simulink model "BIM_3phaseModel_MidInject_DPNV"  (R2022b)
settings: Solver=VariableStepAuto  StartTime=0.0  StopTime=3  RelTol=1e-3
values from neighbouring files (symbols this model uses):
  Ad_s1_s = 0.730402691048646    (= 0.730402691049)    [BIM_init.m]
  Ad_t_s = 0.881911378298176    (= 0.881911378298)    [BIM_init.m]
  Ap_s1_s = 0.975904794542392    (= 0.975904794542)    [BIM_init.m]
  Ap_t_s = 0.995669127615556    (= 0.995669127616)    [BIM_init.m]
  Bd_s1_s = 0.269597308951354    (= 0.269597308951)    [BIM_init.m]
  Bd_t_s = 0.118088621701824    (= 0.118088621702)    [BIM_init.m]
  Bp_s1_s = 0.269597308951354    (= 0.269597308951)    [BIM_init.m]
  Bp_t_s = 0.118088621701824    (= 0.118088621702)    [BIM_init.m]
  Ctr_v_Ki = Ctr_v_Kp*0.1    (= 0.1)    [BIM_init.m]
  Ctr_v_Kp = 1    [BIM_init.m]
  L_m = 5.02e-3    (= 0.00502)    [BIM_init.m]
  L_r = L_m + L_sigma_r    (= 0.00576)    [BIM_init.m]
  m_rotor = 1.5    [BIM_init.m]
  PolePair = 1    [BIM_init.m]
  r_s1_s = 2*R_s    (= 1)    [BIM_init.m]
  r_t_s = R_s/2    (= 0.25)    [BIM_init.m]
  T = 1/fsw    (= 0.0001)    [BIM_init.m]
  tau_r = 0.012255319148936    (= 0.0122553191489)    [BIM_init.m]
  Ts = 1/fsw    (= 0.0001)    [BIM_init.m]
undefined symbols (not defined in the file or in its folder): plecs, sigbuilder_block
libraries: spsabctodq0Lib x8, spsdq0toabcLib x4
(part 1 of 2)
settings Model: Creator=Zhouzhou  LastModifiedBy=Zhouzhou
settings SolverCC: AlgebraicLoopSolver=TrustRegion
settings DebuggingCC: UnconnectedInputMsg=warning  UnconnectedOutputMsg=warning  UnconnectedLineMsg=warning  SFMachineParentedDataDiag=warning
settings ModelReferenceCC: EnableRefExpFcnMdlSchedulingChecks=on
settings RTWCC: DLArmComputeVersion=19.05

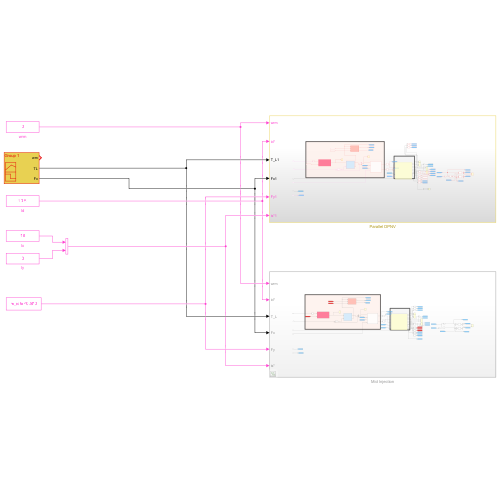
[thumbnail: Simulink's stored preview of the top-level diagram]
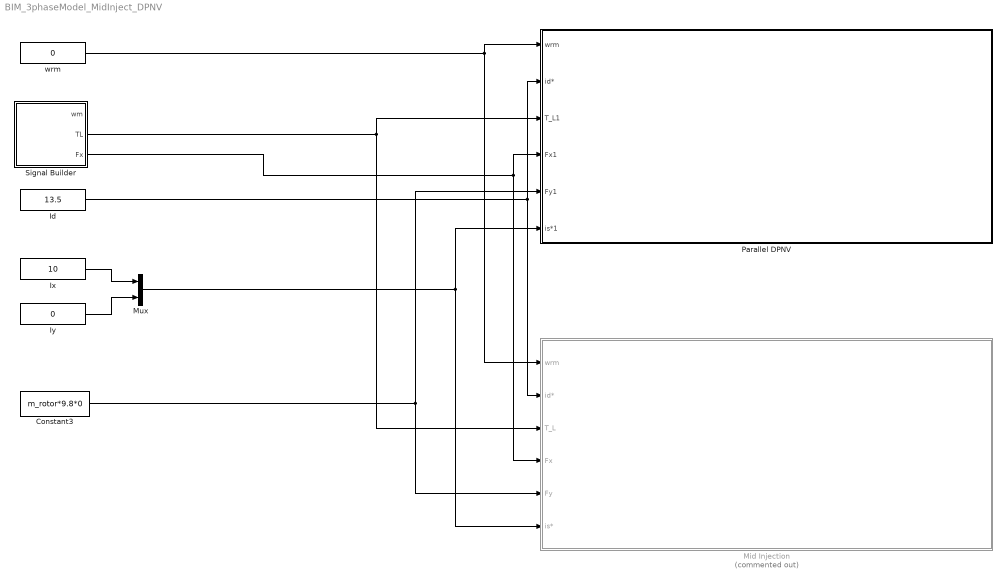
== system BIM_3phaseModel_MidInject_DPNV ==
  Constant3 : Constant  Value=m_rotor*9.8*0
  Id : Constant  Value=13.5
  Ix : Constant  Value=10
  Iy : Constant  Value=0
  Mid Injection : Subsystem  Commented=on
  Mux : Mux  Inputs=2
  Parallel DPNV : Subsystem
  Signal Builder : Subsystem  Tag=STV Subsys  LoadFcn=sigbuilder_block('load');  StartFcn=sigbuilder_block('start');  StopFcn=sigbuilder_block('stop');  ClipboardFcn=sigbuilder_block('clipboard');  mask(Sigbuilder block){tuvar=[0:10]}
      mask help: Simulink:masks:SigbuilderBlock_MD
      mask init:
      | if ~strcmp(get_param(bdroot(gcbh),'SimulationStatus'),'stopped') tuvar = sigbuilder_block('maskInit'); end
      settings: CopyFcn=sigbuilder_block('copy');  DeleteFcn=sigbuilder_block('delete');  ModelCloseFcn=sigbuilder_block('modelClose');  PreSaveFcn=sigbuilder_block('preSave');  PauseFcn=sigbuilder_block('pause');  ContinueFcn=sigbuilder_block('continue');  NameChangeFcn=sigbuilder_block('namechange');  OpenFcn=sigbuilder_block('open',[4.5 4.5 951 480.25 ]);  CloseFcn=sigbuilder_block('close');
      mask Display: plot(0, 0, 100, 100,[2, 2, 32, 32, 2], [68, 8, 8, 68, 68],[32, 2], [38, 38], [32, 19, 2],[53, 60, 44], [32, 17, 17, 2],[16, 16, 31, 31]);txt = getActiveGroup(gcbh);text(2, 100, txt,'verticalAlignment', 'top');
  wrm : Constant  Value=0
  wires:
  wrm/1 -> Mid Injection/1(wrm), Parallel DPNV/1(wrm)
  Signal Builder/2(TL) -> Parallel DPNV/3(T_L1), Mid Injection/3(T_L)
  Id/1 -> Parallel DPNV/2(id*), Mid Injection/2(id*)
  Constant3/1 -> Mid Injection/5(Fy), Parallel DPNV/5(Fy1)
  Signal Builder/3(Fx) -> Parallel DPNV/4(Fx1), Mid Injection/4(Fx)
  Ix/1 -> Mux/1
  Iy/1 -> Mux/2
  Mux/1 -> Mid Injection/6(is*), Parallel DPNV/6(is*1)

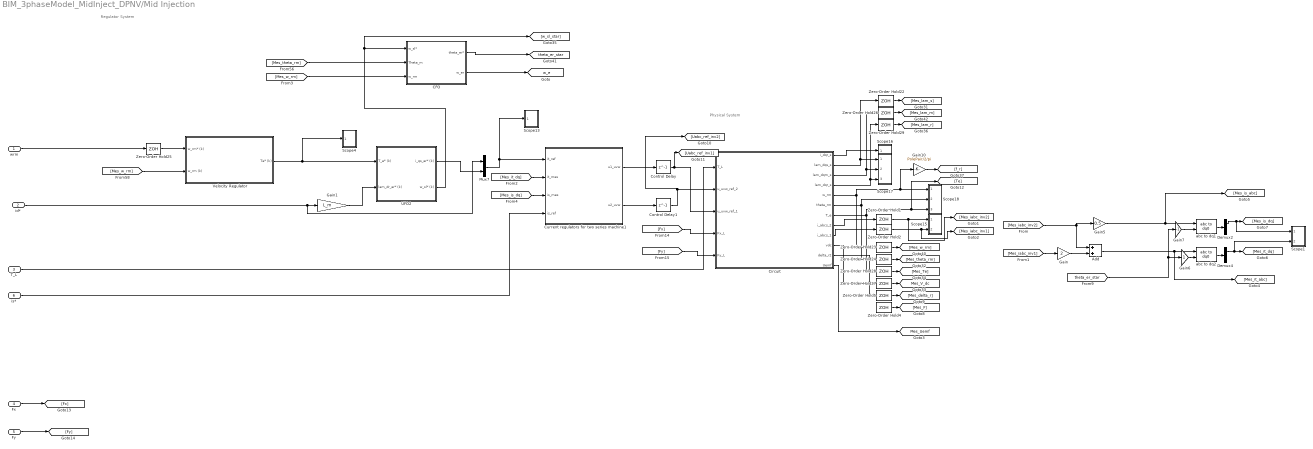
== system BIM_3phaseModel_MidInject_DPNV/Mid Injection ==
  note: Regulator System
  note: Physical System
  wrm : Inport
  id* : Inport  Port=2
  T_L : Inport  Port=3
  Fx : Inport  Port=4
  Fy : Inport  Port=5
  is* : Inport  Port=6
  Add : Sum
  CFO : Subsystem
  Circuit : Subsystem  LoadFcn=plecs('sl', 200);  InitFcn=plecs('sl', 214);  StartFcn=plecs('sl', 208);  StopFcn=plecs('sl', 209);  mask(PlecsCircuit){PLECSData=<binary blob, 27032 chars, not shown>}
      mask prompts: PLECSData "PLECS Data (Do not delete or modify!)"
      mask init:
      | % PLACE CUSTOM INITIALIZATIONS ABOVE
      | % DO NOT REMOVE
      | plecs('sl', 215);
      | % DO NOT REMOVE
      settings: CopyFcn=plecs('sl', 203);  DeleteFcn=plecs('sl', 205);  UndoDeleteFcn=plecs('sl', 206);  PreSaveFcn=plecs('sl', 211);  PostSaveFcn=plecs('sl', 201);  NameChangeFcn=plecs('sl', 210);  DestroyFcn=plecs('sl', 207);  PreCopyFcn=plecs('sl', 216);  OpenFcn=plecs('sl', 202);  ErrorFcn=plerrorfcn
      mask Help: web(['file:///' fullfile(plecsdoc, 'creatingacircuit.html')])
      mask Display: disp('IM Drive System');
  Control Delay : Delay  DelayLength=1  InitialCondition=0  SampleTime=T
  Control Delay1 : Delay  DelayLength=1  InitialCondition=0  SampleTime=T
  Current regulators for two series machine1 : Subsystem
  Demux2 : Demux  Outputs=[2 1]
  Demux4 : Demux  Outputs=[2 1]
  Gain : Gain  Gain=2
  Gain1 : Gain  Gain=L_m
  Gain10 : Gain  Gain=PolePair/2/pi
  Gain5 : Gain  Gain=0.5
  Gain6 : Gain
  Gain7 : Gain  Gain=-1
  Mux7 : Mux  Inputs=2
  Scope1 : Subsystem  LoadFcn=plecs('sl', 300);  InitFcn=plecs('sl', 314);  StartFcn=plecs('sl', 308);  StopFcn=plecs('sl', 309);  mask{Settings=<binary blob, 232 chars, not shown>}
      mask init:
      | plecs('sl', 315);
      settings: CopyFcn=plecs('sl', 303);  DeleteFcn=plecs('sl', 305);  UndoDeleteFcn=plecs('sl', 306);  PreSaveFcn=plecs('sl', 311);  NameChangeFcn=plecs('sl', 310);  DestroyFcn=plecs('sl', 307);  OpenFcn=plecs('sl', 302);  ErrorFcn=plerrorfcn
      mask Display: plot([0.1 0.9 0.9 0.1 0.1], [0.9 0.9 0.5 0.5 0.9])
  Scope13 : Subsystem  LoadFcn=plecs('sl', 300);  InitFcn=plecs('sl', 314);  StartFcn=plecs('sl', 308);  StopFcn=plecs('sl', 309);  mask{Settings=<binary blob, 232 chars, not shown>}
      mask init:
      | plecs('sl', 315);
      settings: CopyFcn=plecs('sl', 303);  DeleteFcn=plecs('sl', 305);  UndoDeleteFcn=plecs('sl', 306);  PreSaveFcn=plecs('sl', 311);  NameChangeFcn=plecs('sl', 310);  DestroyFcn=plecs('sl', 307);  OpenFcn=plecs('sl', 302);  ErrorFcn=plerrorfcn
      mask Display: plot([0.1 0.9 0.9 0.1 0.1], [0.9 0.9 0.5 0.5 0.9])
  Scope15 : Subsystem  LoadFcn=plecs('sl', 300);  InitFcn=plecs('sl', 314);  StartFcn=plecs('sl', 308);  StopFcn=plecs('sl', 309);  mask{Settings=<binary blob, 232 chars, not shown>}
      mask init:
      | plecs('sl', 315);
      settings: CopyFcn=plecs('sl', 303);  DeleteFcn=plecs('sl', 305);  UndoDeleteFcn=plecs('sl', 306);  PreSaveFcn=plecs('sl', 311);  NameChangeFcn=plecs('sl', 310);  DestroyFcn=plecs('sl', 307);  OpenFcn=plecs('sl', 302);  ErrorFcn=plerrorfcn
      mask Display: plot([0.1 0.9 0.9 0.1 0.1], [0.9 0.9 0.5 0.5 0.9])
  Scope16 : Subsystem  LoadFcn=plecs('sl', 300);  InitFcn=plecs('sl', 314);  StartFcn=plecs('sl', 308);  StopFcn=plecs('sl', 309);  mask{Settings=<binary blob, 232 chars, not shown>}
      mask init:
      | plecs('sl', 315);
      settings: CopyFcn=plecs('sl', 303);  DeleteFcn=plecs('sl', 305);  UndoDeleteFcn=plecs('sl', 306);  PreSaveFcn=plecs('sl', 311);  NameChangeFcn=plecs('sl', 310);  DestroyFcn=plecs('sl', 307);  OpenFcn=plecs('sl', 302);  ErrorFcn=plerrorfcn
      mask Display: plot([0.1 0.9 0.9 0.1 0.1], [0.9 0.9 0.5 0.5 0.9])
  Scope17 : Subsystem  LoadFcn=plecs('sl', 300);  InitFcn=plecs('sl', 314);  StartFcn=plecs('sl', 308);  StopFcn=plecs('sl', 309);  mask{Settings=<binary blob, 232 chars, not shown>}
      mask init:
      | plecs('sl', 315);
      settings: CopyFcn=plecs('sl', 303);  DeleteFcn=plecs('sl', 305);  UndoDeleteFcn=plecs('sl', 306);  PreSaveFcn=plecs('sl', 311);  NameChangeFcn=plecs('sl', 310);  DestroyFcn=plecs('sl', 307);  OpenFcn=plecs('sl', 302);  ErrorFcn=plerrorfcn
      mask Display: plot([0.1 0.9 0.9 0.1 0.1], [0.9 0.9 0.5 0.5 0.9])
  Scope18 : Subsystem  LoadFcn=plecs('sl', 300);  InitFcn=plecs('sl', 314);  StartFcn=plecs('sl', 308);  StopFcn=plecs('sl', 309);  mask{Settings=<binary blob, 232 chars, not shown>}
      mask init:
      | plecs('sl', 315);
      settings: CopyFcn=plecs('sl', 303);  DeleteFcn=plecs('sl', 305);  UndoDeleteFcn=plecs('sl', 306);  PreSaveFcn=plecs('sl', 311);  NameChangeFcn=plecs('sl', 310);  DestroyFcn=plecs('sl', 307);  OpenFcn=plecs('sl', 302);  ErrorFcn=plerrorfcn
      mask Display: plot([0.1 0.9 0.9 0.1 0.1], [0.9 0.9 0.5 0.5 0.9])
  Scope4 : Subsystem  LoadFcn=plecs('sl', 300);  InitFcn=plecs('sl', 314);  StartFcn=plecs('sl', 308);  StopFcn=plecs('sl', 309);  mask{Settings=<binary blob, 232 chars, not shown>}
      mask init:
      | plecs('sl', 315);
      settings: CopyFcn=plecs('sl', 303);  DeleteFcn=plecs('sl', 305);  UndoDeleteFcn=plecs('sl', 306);  PreSaveFcn=plecs('sl', 311);  NameChangeFcn=plecs('sl', 310);  DestroyFcn=plecs('sl', 307);  OpenFcn=plecs('sl', 302);  ErrorFcn=plerrorfcn
      mask Display: plot([0.1 0.9 0.9 0.1 0.1], [0.9 0.9 0.5 0.5 0.9])
  UFO2 : Subsystem
  Velocity Regulator : Subsystem
  Zero-Order Hold{1..2,4..5,22..29} (12 alike) : ZeroOrderHold  SampleTime=T
  abc to dq1 : spsabctodq0Lib/abc to dq0  Alignment=Aligned with phase A axis
  abc to dq2 : spsabctodq0Lib/abc to dq0  Alignment=Aligned with phase A axis
  tag scope: Mes_Uemf=global, Mes_V_dc=global, theta_er_star=global, w_e=global
  wires:
  Zero-Order Hold22/1 -> [Mes_lam_s]
  Gain6/1 -> abc to dq2/2
  [theta_er_star] -> Gain7/1, Gain6/1
  [Mes_w_rm] -> CFO/3(w_rm)
  Circuit/5(w_rm) -> Scope18/1(1), Gain10/1, Zero-Order Hold23/1
  Zero-Order Hold29/1 -> [Mes_lam_r]
  Circuit/1(i_dqr_s) -> Scope16/1(1)
  Circuit/6(theta_rm) -> Scope18/2(2), Zero-Order Hold24/1
  CFO/1(theta_er*) -> [theta_er_star]
  Circuit/4(lam_dqr_s) -> Scope17/3(3), Zero-Order Hold29/1
  abc to dq1/1 -> Demux2/1
  Add/1 -> [Mes_it_abc], abc to dq2/1
  UFO2/2(w_sl* (k)) -> [w_sl_star], CFO/1(w_sl*)
  [Mes_iabc_inv1] -> Gain/1
  Demux4/1 -> Scope1/2(2), [Mes_it_dq]
  Mux7/1 -> Current regulators for two series machine1/1(it_ref), Scope13/1(1)
  [Fx] -> Circuit/4(Fx_L)
  [Mes_w_rm] -> Velocity Regulator/2(w_rm (k))
  Circuit/2(lam_dqs_s) -> Scope17/1(1), Zero-Order Hold22/1
  Circuit/7(T_e) -> [Te], Scope18/3(3), Zero-Order Hold28/1
  [Mes_theta_rm] -> CFO/2(Theta_m)
  Current regulators for two series machine1/1(u1_uvw) -> Control Delay/1
  Zero-Order Hold28/1 -> [Mes_Te]
  Gain10/1 -> [f_r]
  Zero-Order Hold4/1 -> [Mes_F]
  id*/1 -> Mux7/1, Gain1/1
  Zero-Order Hold2/1 -> [Mes_iabc_inv1], Scope15/2(2)
  [Mes_iabc_inv2] -> Gain5/1, Add/1
  Zero-Order Hold25/1 -> Velocity Regulator/1(w_rm* (k))
  Current regulators for two series machine1/2(u2_uvw) -> Control Delay1/1
  Gain1/1 -> UFO2/2(lam_dr_er* (k))
  Circuit/8(i_abcs_2) -> Zero-Order Hold1/1
  [Mes_is_dq] -> Current regulators for two series machine1/3(is_mes)
  Circuit/9(i_abcs_1) -> Zero-Order Hold2/1
  Gain/1 -> Add/2
  Zero-Order Hold1/1 -> [Mes_iabc_inv2], Scope15/1(1)
  Zero-Order Hold23/1 -> [Mes_w_rm]
  Demux2/1 -> Scope1/1(1), [Mes_is_dq]
  Circuit/11(delta_r2) -> Zero-Order Hold5/1
  abc to dq2/1 -> Demux4/1
  [Mes_it_dq] -> Current regulators for two series machine1/2(it_mes)
  Velocity Regulator/1(Te* (k)) -> Scope4/1(1), UFO2/1(T_e* (k))
  Zero-Order Hold24/1 -> [Mes_theta_rm]
  Zero-Order Hold26/1 -> [Mes_lam_m]
  Zero-Order Hold27/1 -> [Mes_V_dc]
  [Fy] -> Circuit/5(Fy_L)
  Circuit/10(vdc) -> Zero-Order Hold27/1
  Circuit/3(lam_dqm_s) -> Scope17/2(2), Zero-Order Hold26/1
  CFO/2(w_er) -> [w_e]
  UFO2/1(i_qs_er* (k)) -> Mux7/2
  Zero-Order Hold5/1 -> [Mes_delta_r]
  T_L/1 -> Circuit/1(T_L)
  wrm/1 -> Zero-Order Hold25/1
  Control Delay1/1 -> [Uabc_ref_inv2], Circuit/2(u_uvw_ref_2)
  Control Delay/1 -> Circuit/3(u_uvw_ref_1), [Uabc_ref_inv1]
  Gain5/1 -> abc to dq1/1, [Mes_is_abc]
  Circuit/12(Uemf) -> [Mes_Uemf]
  Gain7/1 -> abc to dq1/2
  Fx/1 -> [Fx]
  Fy/1 -> [Fy]
  is*/1 -> Current regulators for two series machine1/4(is_ref)

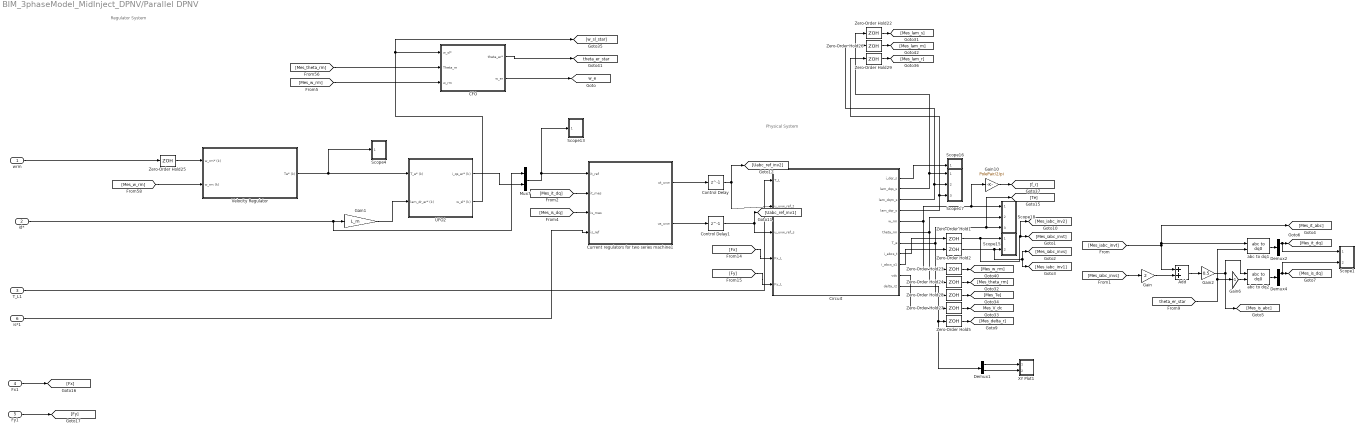
== system BIM_3phaseModel_MidInject_DPNV/Parallel DPNV ==
  note: Physical System
  note: Regulator System
  wrm : Inport
  id* : Inport  Port=2
  T_L1 : Inport  Port=3
  Fx1 : Inport  Port=4
  Fy1 : Inport  Port=5
  is*1 : Inport  Port=6
  Add : Sum
  CFO : Subsystem
  Circuit : Subsystem  LoadFcn=plecs('sl', 200);  InitFcn=plecs('sl', 214);  StartFcn=plecs('sl', 208);  StopFcn=plecs('sl', 209);  mask(PlecsCircuit){PLECSData=<binary blob, 27016 chars, not shown>}
      mask prompts: PLECSData "PLECS Data (Do not delete or modify!)"
      mask init:
      | % PLACE CUSTOM INITIALIZATIONS ABOVE
      | % DO NOT REMOVE
      | plecs('sl', 215);
      | % DO NOT REMOVE
      settings: CopyFcn=plecs('sl', 203);  DeleteFcn=plecs('sl', 205);  UndoDeleteFcn=plecs('sl', 206);  PreSaveFcn=plecs('sl', 211);  PostSaveFcn=plecs('sl', 201);  NameChangeFcn=plecs('sl', 210);  DestroyFcn=plecs('sl', 207);  PreCopyFcn=plecs('sl', 216);  OpenFcn=plecs('sl', 202);  ErrorFcn=plerrorfcn
      mask Help: web(['file:///' fullfile(plecsdoc, 'creatingacircuit.html')])
      mask Display: disp('IM Drive System');
  Control Delay : Delay  DelayLength=1  InitialCondition=0  SampleTime=T
  Control Delay1 : Delay  DelayLength=1  InitialCondition=0  SampleTime=T
  Current regulators for two series machine1 : Subsystem
  Demux1 : Demux  Outputs=2
  Demux2 : Demux  Outputs=[2 1]
  Demux4 : Demux  Outputs=[2 1]
  Gain : Gain  Gain=2
  Gain1 : Gain  Gain=L_m
  Gain10 : Gain  Gain=PolePair/2/pi
  Gain2 : Gain  Gain=0.5
  Gain6 : Gain  Gain=-1
  Mux7 : Mux  Inputs=2
  Scope1 : Subsystem  LoadFcn=plecs('sl', 300);  InitFcn=plecs('sl', 314);  StartFcn=plecs('sl', 308);  StopFcn=plecs('sl', 309);  mask{Settings=<binary blob, 232 chars, not shown>}
      mask init:
      | plecs('sl', 315);
      settings: CopyFcn=plecs('sl', 303);  DeleteFcn=plecs('sl', 305);  UndoDeleteFcn=plecs('sl', 306);  PreSaveFcn=plecs('sl', 311);  NameChangeFcn=plecs('sl', 310);  DestroyFcn=plecs('sl', 307);  OpenFcn=plecs('sl', 302);  ErrorFcn=plerrorfcn
      mask Display: plot([0.1 0.9 0.9 0.1 0.1], [0.9 0.9 0.5 0.5 0.9])
  Scope13 : Subsystem  LoadFcn=plecs('sl', 300);  InitFcn=plecs('sl', 314);  StartFcn=plecs('sl', 308);  StopFcn=plecs('sl', 309);  mask{Settings=<binary blob, 232 chars, not shown>}
      mask init:
      | plecs('sl', 315);
      settings: CopyFcn=plecs('sl', 303);  DeleteFcn=plecs('sl', 305);  UndoDeleteFcn=plecs('sl', 306);  PreSaveFcn=plecs('sl', 311);  NameChangeFcn=plecs('sl', 310);  DestroyFcn=plecs('sl', 307);  OpenFcn=plecs('sl', 302);  ErrorFcn=plerrorfcn
      mask Display: plot([0.1 0.9 0.9 0.1 0.1], [0.9 0.9 0.5 0.5 0.9])
  Scope15 : Subsystem  LoadFcn=plecs('sl', 300);  InitFcn=plecs('sl', 314);  StartFcn=plecs('sl', 308);  StopFcn=plecs('sl', 309);  mask{Settings=<binary blob, 232 chars, not shown>}
      mask init:
      | plecs('sl', 315);
      settings: CopyFcn=plecs('sl', 303);  DeleteFcn=plecs('sl', 305);  UndoDeleteFcn=plecs('sl', 306);  PreSaveFcn=plecs('sl', 311);  NameChangeFcn=plecs('sl', 310);  DestroyFcn=plecs('sl', 307);  OpenFcn=plecs('sl', 302);  ErrorFcn=plerrorfcn
      mask Display: plot([0.1 0.9 0.9 0.1 0.1], [0.9 0.9 0.5 0.5 0.9])
  Scope16 : Subsystem  LoadFcn=plecs('sl', 300);  InitFcn=plecs('sl', 314);  StartFcn=plecs('sl', 308);  StopFcn=plecs('sl', 309);  mask{Settings=<binary blob, 232 chars, not shown>}
      mask init:
      | plecs('sl', 315);
      settings: CopyFcn=plecs('sl', 303);  DeleteFcn=plecs('sl', 305);  UndoDeleteFcn=plecs('sl', 306);  PreSaveFcn=plecs('sl', 311);  NameChangeFcn=plecs('sl', 310);  DestroyFcn=plecs('sl', 307);  OpenFcn=plecs('sl', 302);  ErrorFcn=plerrorfcn
      mask Display: plot([0.1 0.9 0.9 0.1 0.1], [0.9 0.9 0.5 0.5 0.9])
  Scope17 : Subsystem  LoadFcn=plecs('sl', 300);  InitFcn=plecs('sl', 314);  StartFcn=plecs('sl', 308);  StopFcn=plecs('sl', 309);  mask{Settings=<binary blob, 232 chars, not shown>}
      mask init:
      | plecs('sl', 315);
      settings: CopyFcn=plecs('sl', 303);  DeleteFcn=plecs('sl', 305);  UndoDeleteFcn=plecs('sl', 306);  PreSaveFcn=plecs('sl', 311);  NameChangeFcn=plecs('sl', 310);  DestroyFcn=plecs('sl', 307);  OpenFcn=plecs('sl', 302);  ErrorFcn=plerrorfcn
      mask Display: plot([0.1 0.9 0.9 0.1 0.1], [0.9 0.9 0.5 0.5 0.9])
  Scope18 : Subsystem  LoadFcn=plecs('sl', 300);  InitFcn=plecs('sl', 314);  StartFcn=plecs('sl', 308);  StopFcn=plecs('sl', 309);  mask{Settings=<binary blob, 232 chars, not shown>}
      mask init:
      | plecs('sl', 315);
      settings: CopyFcn=plecs('sl', 303);  DeleteFcn=plecs('sl', 305);  UndoDeleteFcn=plecs('sl', 306);  PreSaveFcn=plecs('sl', 311);  NameChangeFcn=plecs('sl', 310);  DestroyFcn=plecs('sl', 307);  OpenFcn=plecs('sl', 302);  ErrorFcn=plerrorfcn
      mask Display: plot([0.1 0.9 0.9 0.1 0.1], [0.9 0.9 0.5 0.5 0.9])
  Scope4 : Subsystem  LoadFcn=plecs('sl', 300);  InitFcn=plecs('sl', 314);  StartFcn=plecs('sl', 308);  StopFcn=plecs('sl', 309);  mask{Settings=<binary blob, 232 chars, not shown>}
      mask init:
      | plecs('sl', 315);
      settings: CopyFcn=plecs('sl', 303);  DeleteFcn=plecs('sl', 305);  UndoDeleteFcn=plecs('sl', 306);  PreSaveFcn=plecs('sl', 311);  NameChangeFcn=plecs('sl', 310);  DestroyFcn=plecs('sl', 307);  OpenFcn=plecs('sl', 302);  ErrorFcn=plerrorfcn
      mask Display: plot([0.1 0.9 0.9 0.1 0.1], [0.9 0.9 0.5 0.5 0.9])
  UFO2 : Subsystem
  Velocity Regulator : Subsystem
  XY Plot1 : Subsystem  LoadFcn=plecs('sl', 317);  InitFcn=plecs('sl', 314);  StartFcn=plecs('sl', 308);  StopFcn=plecs('sl', 309);  mask{Settings=<binary blob, 240 chars, not shown>}
      mask init:
      | plecs('sl', 315);
      settings: CopyFcn=plecs('sl', 318);  DeleteFcn=plecs('sl', 305);  UndoDeleteFcn=plecs('sl', 306);  PreSaveFcn=plecs('sl', 311);  NameChangeFcn=plecs('sl', 310);  DestroyFcn=plecs('sl', 307);  OpenFcn=plecs('sl', 302);  ErrorFcn=plerrorfcn
      mask Display:
      | plot([0.05 0.95 0.95 0.05 0.05], [0.95 0.95 0.05 0.05 0.95])
      | plot(0.5+sin((0:0.2:2)*pi)*0.3, 0.5+sin((0:0.2:2)*pi + pi/4)*0.3);
  Zero-Order Hold{1..2,5,22..29} (11 alike) : ZeroOrderHold  SampleTime=T
  abc to dq1 : spsabctodq0Lib/abc to dq0  Alignment=Aligned with phase A axis
  abc to dq2 : spsabctodq0Lib/abc to dq0  Alignment=Aligned with phase A axis
  tag scope: Mes_V_dc=global, theta_er_star=global, w_e=global
  wires:
  Zero-Order Hold22/1 -> [Mes_lam_s]
  Gain6/1 -> abc to dq2/2
  [theta_er_star] -> Gain6/1, abc to dq1/2
  Circuit/5(w_rm) -> Scope18/1(1), Gain10/1, Zero-Order Hold23/1
  Zero-Order Hold29/1 -> [Mes_lam_r]
  Control Delay/1 -> Circuit/2(u_uvw_ref_t), [Uabc_ref_inv2]
  Circuit/1(i_dqr_s) -> Scope16/1(1)
  Circuit/6(theta_rm) -> Scope18/2(2), Zero-Order Hold24/1
  Circuit/4(lam_dqr_s) -> Scope17/3(3), Zero-Order Hold29/1
  abc to dq1/1 -> Demux2/1
  Gain2/1 -> abc to dq2/1, [Mes_is_abc]
  [Mes_iabc_invs] -> Gain/1
  Demux4/1 -> Scope1/2(2), [Mes_is_dq]
  Circuit/2(lam_dqs_s) -> Scope17/1(1), Zero-Order Hold22/1
  Circuit/7(T_e) -> [Te], Scope18/3(3), Zero-Order Hold28/1
  Current regulators for two series machine1/1(ut_uvw) -> Control Delay/1
  Zero-Order Hold28/1 -> [Mes_Te]
  Gain10/1 -> [f_r]
  Zero-Order Hold2/1 -> [Mes_iabc_invs], [Mes_iabc_inv1], Scope15/2(2)
  [Mes_iabc_invt] -> abc to dq1/1, [Mes_it_abc], Add/1
  Current regulators for two series machine1/2(us_uvw) -> Control Delay1/1
  Circuit/8(i_abcs_t) -> Zero-Order Hold1/1
  [Mes_is_dq] -> Current regulators for two series machine1/3(is_mes)
  Circuit/9(i_abcs_s1) -> Zero-Order Hold2/1
  Gain/1 -> Add/2
  Zero-Order Hold1/1 -> [Mes_iabc_inv2], [Mes_iabc_invt], Scope15/1(1)
  Zero-Order Hold23/1 -> [Mes_w_rm]
  Demux2/1 -> Scope1/1(1), [Mes_it_dq]
  Circuit/11(delta_r2) -> Demux1/1, Zero-Order Hold5/1
  Control Delay1/1 -> Circuit/3(u_uvw_ref_s), [Uabc_ref_inv1]
  abc to dq2/1 -> Demux4/1
  [Mes_it_dq] -> Current regulators for two series machine1/2(it_mes)
  Demux1/2 -> XY Plot1/2(2)
  Demux1/1 -> XY Plot1/1(1)
  Add/1 -> Gain2/1
  Zero-Order Hold24/1 -> [Mes_theta_rm]
  Zero-Order Hold26/1 -> [Mes_lam_m]
  Zero-Order Hold27/1 -> [Mes_V_dc]
  Circuit/10(vdc) -> Zero-Order Hold27/1
  Circuit/3(lam_dqm_s) -> Scope17/2(2), Zero-Order Hold26/1
  Zero-Order Hold5/1 -> [Mes_delta_r]
  [Fy] -> Circuit/5(Fy_L)
  [Fx] -> Circuit/4(Fx_L)
  Fy1/1 -> [Fy]
  [Mes_w_rm] -> Velocity Regulator/2(w_rm (k))
  Velocity Regulator/1(Te* (k)) -> Scope4/1(1), UFO2/1(T_e* (k))
  CFO/1(theta_er*) -> [theta_er_star]
  Fx1/1 -> [Fx]
  wrm/1 -> Zero-Order Hold25/1
  UFO2/1(i_qs_er* (k)) -> Mux7/2
  [Mes_theta_rm] -> CFO/2(Theta_m)
  UFO2/2(w_sl* (k)) -> [w_sl_star], CFO/1(w_sl*)
  Gain1/1 -> UFO2/2(lam_dr_er* (k))
  id*/1 -> Mux7/1, Gain1/1
  Zero-Order Hold25/1 -> Velocity Regulator/1(w_rm* (k))
  T_L1/1 -> Circuit/1(T_L)
  CFO/2(w_er) -> [w_e]
  Mux7/1 -> Scope13/1(1), Current regulators for two series machine1/1(it_ref)
  is*1/1 -> Current regulators for two series machine1/4(is_ref)
  [Mes_w_rm] -> CFO/3(w_rm)

== system BIM_3phaseModel_MidInject_DPNV/Signal Builder ==
  Demux : Demux  Tag=STV Demux  Outputs=3
      settings: DisplayOption=none
  FromWs : FromWorkspace  Tag=STV FromWs  VariableName=tuvar
      SigBuilderData=|
      | common.afterFinalStr = 'Extrapolate'
      | common.sampleTime = 0
      | dataSet.timeRange = [0 10]
      | dataSet.name = 'Group 1'
      | sbobj.Groups.Name = 'Group 1'
      | sbobj.Groups.Signals(1).Name = 'wm'
      | sbobj.Groups.Signals(1).XData = [0 0.25 0.25 10]
      | sbobj.Groups.Signals(1).YData = [0 0 100 100]
      | sbobj.Groups.Signals(2).Name = 'TL'
      | sbobj.Groups.Signals(2).XData = [0 2 2 10]
      | sbobj.Groups.Signals(2).YData = [0 0 1.17 1.17]
      | sbobj.Groups.Signals(3).Name = 'Fx'
      | sbobj.Groups.Signals(3).XData = [0 2.25 2.25 10]
      | sbobj.Groups.Signals(3).YData = [0 0 10 10]
  wm : Outport  Tag=STV Outport
  TL : Outport  Tag=STV Outport  Port=2
  Fx : Outport  Tag=STV Outport  Port=3
  wires:
  FromWs/1 -> Demux/1
  Demux/1 -> wm/1
  Demux/2 -> TL/1
  Demux/3 -> Fx/1

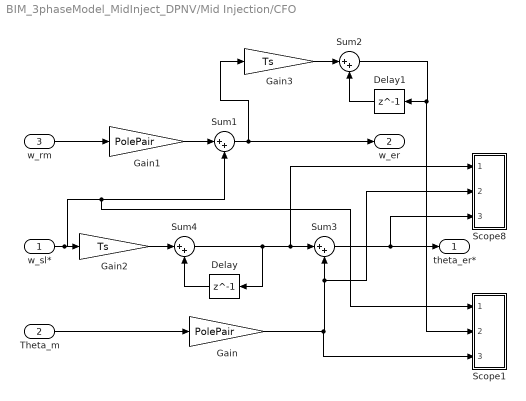
== system BIM_3phaseModel_MidInject_DPNV/Mid Injection/CFO ==
  w_sl* : Inport
  Theta_m : Inport  Port=2
  w_rm : Inport  Port=3
  Delay : Delay  DelayLength=1  InitialCondition=0  SampleTime=Ts
  Delay1 : Delay  DelayLength=1  InitialCondition=0  SampleTime=Ts
  Gain : Gain  Gain=PolePair
  Gain1 : Gain  Gain=PolePair
  Gain2 : Gain  Gain=Ts
  Gain3 : Gain  Gain=Ts
  Scope1 : Subsystem  LoadFcn=plecs('sl', 300);  InitFcn=plecs('sl', 314);  StartFcn=plecs('sl', 308);  StopFcn=plecs('sl', 309);  mask{Settings=<binary blob, 232 chars, not shown>}
      mask init:
      | plecs('sl', 315);
      settings: CopyFcn=plecs('sl', 303);  DeleteFcn=plecs('sl', 305);  UndoDeleteFcn=plecs('sl', 306);  PreSaveFcn=plecs('sl', 311);  NameChangeFcn=plecs('sl', 310);  DestroyFcn=plecs('sl', 307);  OpenFcn=plecs('sl', 302);  ErrorFcn=plerrorfcn
      mask Display: plot([0.1 0.9 0.9 0.1 0.1], [0.9 0.9 0.5 0.5 0.9])
  Scope8 : Subsystem  LoadFcn=plecs('sl', 300);  InitFcn=plecs('sl', 314);  StartFcn=plecs('sl', 308);  StopFcn=plecs('sl', 309);  mask{Settings=<binary blob, 232 chars, not shown>}
      mask init:
      | plecs('sl', 315);
      settings: CopyFcn=plecs('sl', 303);  DeleteFcn=plecs('sl', 305);  UndoDeleteFcn=plecs('sl', 306);  PreSaveFcn=plecs('sl', 311);  NameChangeFcn=plecs('sl', 310);  DestroyFcn=plecs('sl', 307);  OpenFcn=plecs('sl', 302);  ErrorFcn=plerrorfcn
      mask Display: plot([0.1 0.9 0.9 0.1 0.1], [0.9 0.9 0.5 0.5 0.9])
  Sum{1..4} (4 alike) : Sum  Inputs=|++
  theta_er* : Outport
  w_er : Outport  Port=2
  wires:
  Theta_m/1 -> Gain/1
  Sum4/1 -> Scope8/1(1), Sum3/1, Delay/1
  Sum3/1 -> Scope8/3(3), theta_er*/1
  w_sl*/1 -> Scope1/1(1), Sum1/2, Gain2/1
  Gain/1 -> Scope1/3(3), Scope8/2(2), Sum3/2
  Delay/1 -> Sum4/2
  Gain2/1 -> Sum4/1
  w_rm/1 -> Gain1/1
  Gain1/1 -> Sum1/1
  Delay1/1 -> Sum2/2
  Sum1/1 -> Gain3/1, w_er/1
  Gain3/1 -> Sum2/1
  Sum2/1 -> Scope1/2(2), Delay1/1

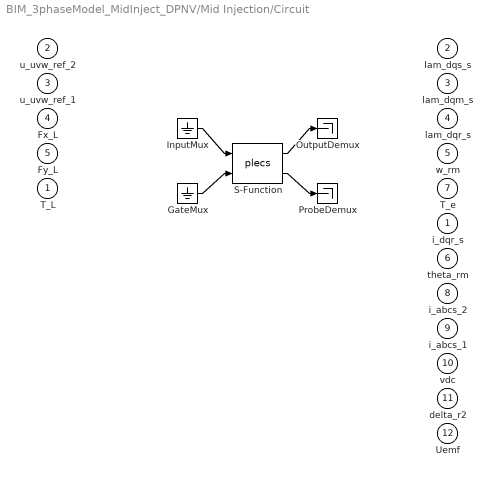
== system BIM_3phaseModel_MidInject_DPNV/Mid Injection/Circuit ==
  T_L : Inport  PortDimensions=1
  u_uvw_ref_2 : Inport  Port=2  PortDimensions=3
  u_uvw_ref_1 : Inport  Port=3  PortDimensions=3
  Fx_L : Inport  Port=4  PortDimensions=1
  Fy_L : Inport  Port=5  PortDimensions=1
  " GateMux " : Ground
  " InputMux " : Ground
  " OutputDemux " : Terminator
  " ProbeDemux " : Terminator
  " S-Function " : S-Function  FunctionName=plecs  SFunctionDeploymentMode=off  EnableBusSupport=off
  i_dqr_s : Outport  PortDimensions=3
  lam_dqs_s : Outport  Port=2  PortDimensions=2
  lam_dqm_s : Outport  Port=3  PortDimensions=2
  lam_dqr_s : Outport  Port=4  PortDimensions=2
  w_rm : Outport  Port=5  PortDimensions=1
  theta_rm : Outport  Port=6  PortDimensions=1
  T_e : Outport  Port=7  PortDimensions=1
  i_abcs_2 : Outport  Port=8  PortDimensions=3
  i_abcs_1 : Outport  Port=9  PortDimensions=3
  vdc : Outport  Port=10  PortDimensions=1
  delta_r2 : Outport  Port=11  PortDimensions=2
  Uemf : Outport  Port=12  PortDimensions=3
  wires:
  " InputMux "/1 -> " S-Function "/1
  " GateMux "/1 -> " S-Function "/2
  " S-Function "/1 -> " OutputDemux "/1
  " S-Function "/2 -> " ProbeDemux "/1

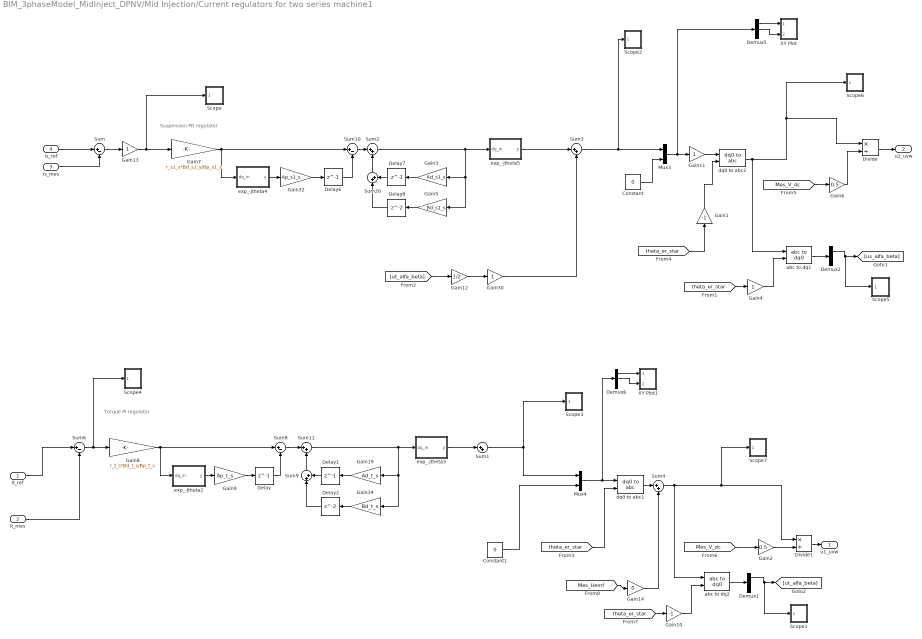
== system BIM_3phaseModel_MidInject_DPNV/Mid Injection/Current regulators for two series machine1 ==
  note: Suspension PR regulator
  note: Torque PI regulator
  it_ref : Inport  PortDimensions=2
  it_mes : Inport  Port=2  PortDimensions=2
  is_mes : Inport  Port=3  PortDimensions=2
  is_ref : Inport  Port=4  PortDimensions=2
  Constant : Constant  Value=0
  Constant1 : Constant  Value=0
  Delay{,1,6..7} (4 alike) : Delay  DelayLength=1  SampleTime=Ts
  Delay2 : Delay  SampleTime=Ts
  Delay8 : Delay  SampleTime=Ts
  Demux1 : Demux  Outputs=[2 1]
  Demux2 : Demux  Outputs=[2 1]
  Demux5 : Demux  Outputs=3
  Demux6 : Demux  Outputs=3
  Divide : Product  Inputs=*/
  Divide1 : Product  Inputs=*/
  Gain1 : Gain  Gain=-1
  Gain10 : Gain  Gain=-1
  Gain{4,11,13,30} (4 alike) : Gain
  Gain12 : Gain  Gain=1/2
  Gain14 : Gain  Gain=0
  Gain19 : Gain  Gain=Ad_t_s
  Gain2 : Gain  Gain=0.5
  Gain3 : Gain  Gain=Ad_s1_s
  Gain32 : Gain  Gain=Ap_s1_s
  Gain34 : Gain  Gain=Bd_t_s
  Gain5 : Gain  Gain=Bd_s1_s
  Gain6 : Gain  Gain=0.5
  Gain7 : Gain  Gain=r_s1_s*Bd_s1_s/Bp_s1_s
  Gain8 : Gain  Gain=r_t_s*Bd_t_s/Bp_t_s
  Gain9 : Gain  Gain=Ap_t_s
  Mux3 : Mux  Inputs=[2 1]
  Mux4 : Mux  Inputs=[2 1]
  Scope : Subsystem  LoadFcn=plecs('sl', 300);  InitFcn=plecs('sl', 314);  StartFcn=plecs('sl', 308);  StopFcn=plecs('sl', 309);  mask{Settings=<binary blob, 232 chars, not shown>}
      mask init:
      | plecs('sl', 315);
      settings: CopyFcn=plecs('sl', 303);  DeleteFcn=plecs('sl', 305);  UndoDeleteFcn=plecs('sl', 306);  PreSaveFcn=plecs('sl', 311);  NameChangeFcn=plecs('sl', 310);  DestroyFcn=plecs('sl', 307);  OpenFcn=plecs('sl', 302);  ErrorFcn=plerrorfcn
      mask Display: plot([0.1 0.9 0.9 0.1 0.1], [0.9 0.9 0.5 0.5 0.9])
  Scope1 : Subsystem  LoadFcn=plecs('sl', 300);  InitFcn=plecs('sl', 314);  StartFcn=plecs('sl', 308);  StopFcn=plecs('sl', 309);  mask{Settings=<binary blob, 232 chars, not shown>}
      mask init:
      | plecs('sl', 315);
      settings: CopyFcn=plecs('sl', 303);  DeleteFcn=plecs('sl', 305);  UndoDeleteFcn=plecs('sl', 306);  PreSaveFcn=plecs('sl', 311);  NameChangeFcn=plecs('sl', 310);  DestroyFcn=plecs('sl', 307);  OpenFcn=plecs('sl', 302);  ErrorFcn=plerrorfcn
      mask Display: plot([0.1 0.9 0.9 0.1 0.1], [0.9 0.9 0.5 0.5 0.9])
  Scope2 : Subsystem  LoadFcn=plecs('sl', 300);  InitFcn=plecs('sl', 314);  StartFcn=plecs('sl', 308);  StopFcn=plecs('sl', 309);  mask{Settings=<binary blob, 232 chars, not shown>}
      mask init:
      | plecs('sl', 315);
      settings: CopyFcn=plecs('sl', 303);  DeleteFcn=plecs('sl', 305);  UndoDeleteFcn=plecs('sl', 306);  PreSaveFcn=plecs('sl', 311);  NameChangeFcn=plecs('sl', 310);  DestroyFcn=plecs('sl', 307);  OpenFcn=plecs('sl', 302);  ErrorFcn=plerrorfcn
      mask Display: plot([0.1 0.9 0.9 0.1 0.1], [0.9 0.9 0.5 0.5 0.9])
  Scope3 : Subsystem  LoadFcn=plecs('sl', 300);  InitFcn=plecs('sl', 314);  StartFcn=plecs('sl', 308);  StopFcn=plecs('sl', 309);  mask{Settings=<binary blob, 232 chars, not shown>}
      mask init:
      | plecs('sl', 315);
      settings: CopyFcn=plecs('sl', 303);  DeleteFcn=plecs('sl', 305);  UndoDeleteFcn=plecs('sl', 306);  PreSaveFcn=plecs('sl', 311);  NameChangeFcn=plecs('sl', 310);  DestroyFcn=plecs('sl', 307);  OpenFcn=plecs('sl', 302);  ErrorFcn=plerrorfcn
      mask Display: plot([0.1 0.9 0.9 0.1 0.1], [0.9 0.9 0.5 0.5 0.9])
  Scope4 : Subsystem  LoadFcn=plecs('sl', 300);  InitFcn=plecs('sl', 314);  StartFcn=plecs('sl', 308);  StopFcn=plecs('sl', 309);  mask{Settings=<binary blob, 232 chars, not shown>}
      mask init:
      | plecs('sl', 315);
      settings: CopyFcn=plecs('sl', 303);  DeleteFcn=plecs('sl', 305);  UndoDeleteFcn=plecs('sl', 306);  PreSaveFcn=plecs('sl', 311);  NameChangeFcn=plecs('sl', 310);  DestroyFcn=plecs('sl', 307);  OpenFcn=plecs('sl', 302);  ErrorFcn=plerrorfcn
      mask Display: plot([0.1 0.9 0.9 0.1 0.1], [0.9 0.9 0.5 0.5 0.9])
  Scope5 : Subsystem  LoadFcn=plecs('sl', 300);  InitFcn=plecs('sl', 314);  StartFcn=plecs('sl', 308);  StopFcn=plecs('sl', 309);  mask{Settings=<binary blob, 232 chars, not shown>}
      mask init:
      | plecs('sl', 315);
      settings: CopyFcn=plecs('sl', 303);  DeleteFcn=plecs('sl', 305);  UndoDeleteFcn=plecs('sl', 306);  PreSaveFcn=plecs('sl', 311);  NameChangeFcn=plecs('sl', 310);  DestroyFcn=plecs('sl', 307);  OpenFcn=plecs('sl', 302);  ErrorFcn=plerrorfcn
      mask Display: plot([0.1 0.9 0.9 0.1 0.1], [0.9 0.9 0.5 0.5 0.9])
  Scope6 : Subsystem  LoadFcn=plecs('sl', 300);  InitFcn=plecs('sl', 314);  StartFcn=plecs('sl', 308);  StopFcn=plecs('sl', 309);  mask{Settings=<binary blob, 232 chars, not shown>}
      mask init:
      | plecs('sl', 315);
      settings: CopyFcn=plecs('sl', 303);  DeleteFcn=plecs('sl', 305);  UndoDeleteFcn=plecs('sl', 306);  PreSaveFcn=plecs('sl', 311);  NameChangeFcn=plecs('sl', 310);  DestroyFcn=plecs('sl', 307);  OpenFcn=plecs('sl', 302);  ErrorFcn=plerrorfcn
      mask Display: plot([0.1 0.9 0.9 0.1 0.1], [0.9 0.9 0.5 0.5 0.9])
  Scope7 : Subsystem  LoadFcn=plecs('sl', 300);  InitFcn=plecs('sl', 314);  StartFcn=plecs('sl', 308);  StopFcn=plecs('sl', 309);  mask{Settings=<binary blob, 232 chars, not shown>}
      mask init:
      | plecs('sl', 315);
      settings: CopyFcn=plecs('sl', 303);  DeleteFcn=plecs('sl', 305);  UndoDeleteFcn=plecs('sl', 306);  PreSaveFcn=plecs('sl', 311);  NameChangeFcn=plecs('sl', 310);  DestroyFcn=plecs('sl', 307);  OpenFcn=plecs('sl', 302);  ErrorFcn=plerrorfcn
      mask Display: plot([0.1 0.9 0.9 0.1 0.1], [0.9 0.9 0.5 0.5 0.9])
  Sum{,6,8,10} (4 alike) : Sum  Inputs=|+-
  Sum{1..4,9,11,20} (7 alike) : Sum  Inputs=|++
  XY Plot : Subsystem  LoadFcn=plecs('sl', 317);  InitFcn=plecs('sl', 314);  StartFcn=plecs('sl', 308);  StopFcn=plecs('sl', 309);  mask{Settings=<binary blob, 240 chars, not shown>}
      mask init:
      | plecs('sl', 315);
      settings: CopyFcn=plecs('sl', 318);  DeleteFcn=plecs('sl', 305);  UndoDeleteFcn=plecs('sl', 306);  PreSaveFcn=plecs('sl', 311);  NameChangeFcn=plecs('sl', 310);  DestroyFcn=plecs('sl', 307);  OpenFcn=plecs('sl', 302);  ErrorFcn=plerrorfcn
      mask Display:
      | plot([0.05 0.95 0.95 0.05 0.05], [0.95 0.95 0.05 0.05 0.95])
      | plot(0.5+sin((0:0.2:2)*pi)*0.3, 0.5+sin((0:0.2:2)*pi + pi/4)*0.3);
  XY Plot1 : Subsystem  LoadFcn=plecs('sl', 317);  InitFcn=plecs('sl', 314);  StartFcn=plecs('sl', 308);  StopFcn=plecs('sl', 309);  mask{Settings=<binary blob, 240 chars, not shown>}
      mask init:
      | plecs('sl', 315);
      settings: CopyFcn=plecs('sl', 318);  DeleteFcn=plecs('sl', 305);  UndoDeleteFcn=plecs('sl', 306);  PreSaveFcn=plecs('sl', 311);  NameChangeFcn=plecs('sl', 310);  DestroyFcn=plecs('sl', 307);  OpenFcn=plecs('sl', 302);  ErrorFcn=plerrorfcn
      mask Display:
      | plot([0.05 0.95 0.95 0.05 0.05], [0.95 0.95 0.05 0.05 0.95])
      | plot(0.5+sin((0:0.2:2)*pi)*0.3, 0.5+sin((0:0.2:2)*pi + pi/4)*0.3);
  abc to dq1 : spsabctodq0Lib/abc to dq0  Alignment=Aligned with phase A axis
  abc to dq2 : spsabctodq0Lib/abc to dq0  Alignment=Aligned with phase A axis
  dq0 to abc1 : spsdq0toabcLib/dq0 to abc  Alignment=Aligned with phase A axis
  dq0 to abc2 : spsdq0toabcLib/dq0 to abc  Alignment=Aligned with phase A axis
  exp_-jtheta2 : Subsystem
  exp_-jtheta3 : Subsystem
  exp_-jtheta4 : Subsystem
  exp_-jtheta5 : Subsystem
  u1_uvw : Outport  PortDimensions=3
  u2_uvw : Outport  Port=2  PortDimensions=3
  wires:
  Sum6/1 -> Scope4/1(1), Gain8/1
  Mux3/1 -> Gain11/1, Demux5/1
  dq0 to abc2/1 -> abc to dq1/1, Divide/1, Scope6/1(1)
  Sum11/1 -> Gain34/1, Gain19/1, exp_-jtheta3/1(dq_in)
  Constant1/1 -> Mux4/2
  Demux5/1 -> XY Plot/1(1)
  Demux5/2 -> XY Plot/2(2)
  Demux6/2 -> XY Plot1/2(2)
  Demux6/1 -> XY Plot1/1(1)
  Constant/1 -> Mux3/2
  Gain8/1 -> Sum8/1, exp_-jtheta2/1(dq_in)
  Gain9/1 -> Delay/1
  Sum8/1 -> Sum11/1
  Delay/1 -> Sum8/2
  Gain19/1 -> Delay1/1
  Gain34/1 -> Delay2/1
  Delay1/1 -> Sum9/2
  Delay2/1 -> Sum9/1
  Sum9/1 -> Sum11/2
  Sum2/1 -> Gain5/1, Gain3/1, exp_-jtheta5/1(dq_in)
  Delay8/1 -> Sum20/1
  Delay7/1 -> Sum20/2
  Delay6/1 -> Sum10/2
  Gain5/1 -> Delay8/1
  Sum20/1 -> Sum2/2
  Gain3/1 -> Delay7/1
  Sum/1 -> Gain13/1
  Gain32/1 -> Delay6/1
  Gain7/1 -> Sum10/1, exp_-jtheta4/1(dq_in)
  Sum10/1 -> Sum2/1
  it_ref/1 -> Sum6/1
  it_mes/1 -> Sum6/2
  exp_-jtheta2/1(y) -> Gain9/1
  [theta_er_star] -> dq0 to abc1/2
  is_ref/1 -> Sum/1
  is_mes/1 -> Sum/2
  exp_-jtheta4/1(y) -> Gain32/1
  [theta_er_star] -> Gain1/1
  Gain1/1 -> dq0 to abc2/2
  abc to dq1/1 -> Demux2/1
  [theta_er_star] -> Gain4/1
  Gain4/1 -> abc to dq1/2
  Demux2/1 -> Scope5/1(1), [us_alfa_beta]
  Gain12/1 -> Gain30/1
  [ut_alfa_beta] -> Gain12/1
  exp_-jtheta3/1(y) -> Sum1/1
  [Mes_V_dc] -> Gain6/1
  Divide/1 -> u2_uvw/1
  [Mes_V_dc] -> Gain2/1
  Divide1/1 -> u1_uvw/1
  Gain2/1 -> Divide1/2
  Gain6/1 -> Divide/2
  Demux1/1 -> Scope1/1(1), [ut_alfa_beta]
  [theta_er_star] -> Gain10/1
  Gain10/1 -> abc to dq2/2
  Sum4/1 -> abc to dq2/1, Scope7/1(1), Divide1/1
  Mux4/1 -> Demux6/1, dq0 to abc1/1
  Sum1/1 -> Mux4/1, Scope3/1(1)
  Sum3/1 -> Scope2/1(1), Mux3/1
  exp_-jtheta5/1(y) -> Sum3/1
  Gain30/1 -> Sum3/2
  Gain11/1 -> dq0 to abc2/1
  Gain13/1 -> Gain7/1, Scope/1(1)
  abc to dq2/1 -> Demux1/1
  dq0 to abc1/1 -> Sum4/1
  [Mes_Uemf] -> Gain14/1
  Gain14/1 -> Sum4/2

== system BIM_3phaseModel_MidInject_DPNV/Mid Injection/Scope1 ==
  1 : Inport
  2 : Inport  Port=2
  " 1 " : DataTypeConversion
  " 2 " : DataTypeConversion
  " InputMux " : Mux  Inputs=2
  " S-Function " : S-Function  FunctionName=plecs  SFunctionDeploymentMode=off  EnableBusSupport=off
  wires:
  " InputMux "/1 -> " S-Function "/1
  1/1 -> " 1 "/1
  " 1 "/1 -> " InputMux "/1
  2/1 -> " 2 "/1
  " 2 "/1 -> " InputMux "/2

== system BIM_3phaseModel_MidInject_DPNV/Mid Injection/Scope13 ==
  1 : Inport
  " 1 " : DataTypeConversion
  " InputMux " : Mux  Inputs=1
  " S-Function " : S-Function  FunctionName=plecs  SFunctionDeploymentMode=off  EnableBusSupport=off
  wires:
  " InputMux "/1 -> " S-Function "/1
  1/1 -> " 1 "/1
  " 1 "/1 -> " InputMux "/1

== system BIM_3phaseModel_MidInject_DPNV/Mid Injection/Scope15 ==
  1 : Inport
  2 : Inport  Port=2
  " 1 " : DataTypeConversion
  " 2 " : DataTypeConversion
  " InputMux " : Mux  Inputs=2
  " S-Function " : S-Function  FunctionName=plecs  SFunctionDeploymentMode=off  EnableBusSupport=off
  wires:
  " InputMux "/1 -> " S-Function "/1
  1/1 -> " 1 "/1
  " 1 "/1 -> " InputMux "/1
  2/1 -> " 2 "/1
  " 2 "/1 -> " InputMux "/2

== system BIM_3phaseModel_MidInject_DPNV/Mid Injection/Scope16 ==
  1 : Inport
  " 1 " : DataTypeConversion
  " InputMux " : Mux  Inputs=1
  " S-Function " : S-Function  FunctionName=plecs  SFunctionDeploymentMode=off  EnableBusSupport=off
  wires:
  " InputMux "/1 -> " S-Function "/1
  1/1 -> " 1 "/1
  " 1 "/1 -> " InputMux "/1

== system BIM_3phaseModel_MidInject_DPNV/Mid Injection/Scope17 ==
  1 : Inport
  2 : Inport  Port=2
  3 : Inport  Port=3
  " 1 " : DataTypeConversion
  " 2 " : DataTypeConversion
  " 3 " : DataTypeConversion
  " InputMux " : Mux  Inputs=3
  " S-Function " : S-Function  FunctionName=plecs  SFunctionDeploymentMode=off  EnableBusSupport=off
  wires:
  " InputMux "/1 -> " S-Function "/1
  1/1 -> " 1 "/1
  " 1 "/1 -> " InputMux "/1
  2/1 -> " 2 "/1
  " 2 "/1 -> " InputMux "/2
  3/1 -> " 3 "/1
  " 3 "/1 -> " InputMux "/3

== system BIM_3phaseModel_MidInject_DPNV/Mid Injection/Scope18 ==
  1 : Inport
  2 : Inport  Port=2
  3 : Inport  Port=3
  " 1 " : DataTypeConversion
  " 2 " : DataTypeConversion
  " 3 " : DataTypeConversion
  " InputMux " : Mux  Inputs=3
  " S-Function " : S-Function  FunctionName=plecs  SFunctionDeploymentMode=off  EnableBusSupport=off
  wires:
  " InputMux "/1 -> " S-Function "/1
  1/1 -> " 1 "/1
  " 1 "/1 -> " InputMux "/1
  2/1 -> " 2 "/1
  " 2 "/1 -> " InputMux "/2
  3/1 -> " 3 "/1
  " 3 "/1 -> " InputMux "/3

== system BIM_3phaseModel_MidInject_DPNV/Mid Injection/Scope4 ==
  1 : Inport
  " 1 " : DataTypeConversion
  " InputMux " : Mux  Inputs=1
  " S-Function " : S-Function  FunctionName=plecs  SFunctionDeploymentMode=off  EnableBusSupport=off
  wires:
  " InputMux "/1 -> " S-Function "/1
  1/1 -> " 1 "/1
  " 1 "/1 -> " InputMux "/1

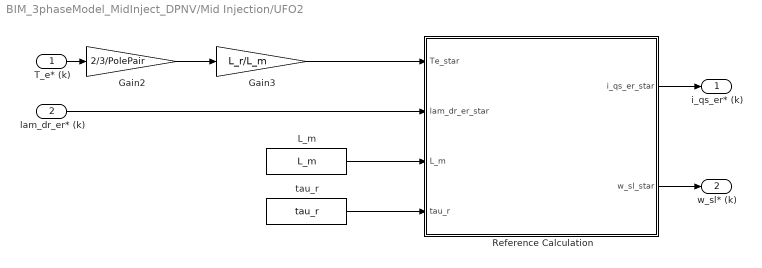
== system BIM_3phaseModel_MidInject_DPNV/Mid Injection/UFO2 ==
  T_e* (k) : Inport
  lam_dr_er* (k) : Inport  Port=2
  Gain2 : Gain  Gain=2/3/PolePair
  Gain3 : Gain  Gain=L_r/L_m
  L_m : Constant  Value=L_m
  Reference Calculation : MATLAB Function  TreatAsAtomicUnit=on
  tau_r : Constant  Value=tau_r
  i_qs_er* (k) : Outport
  w_sl* (k) : Outport  Port=2
  wires:
  lam_dr_er* (k)/1 -> Reference Calculation/2(lam_dr_er_star)
  T_e* (k)/1 -> Gain2/1
  Gain2/1 -> Gain3/1
  Gain3/1 -> Reference Calculation/1(Te_star)
  L_m/1 -> Reference Calculation/3(L_m)
  tau_r/1 -> Reference Calculation/4(tau_r)
  Reference Calculation/2(w_sl_star) -> w_sl* (k)/1
  Reference Calculation/1(i_qs_er_star) -> i_qs_er* (k)/1

== system BIM_3phaseModel_MidInject_DPNV/Mid Injection/Velocity Regulator ==
  w_rm* (k) : Inport
  w_rm (k) : Inport  Port=2
  Rate Limiter : RateLimiter  RisingSlewLimit=50  FallingSlewLimit=-50  SampleTimeMode=inherited
  Scope4 : Subsystem  LoadFcn=plecs('sl', 300);  InitFcn=plecs('sl', 314);  StartFcn=plecs('sl', 308);  StopFcn=plecs('sl', 309);  mask{Settings=<binary blob, 232 chars, not shown>}
      mask init:
      | plecs('sl', 315);
      settings: CopyFcn=plecs('sl', 303);  DeleteFcn=plecs('sl', 305);  UndoDeleteFcn=plecs('sl', 306);  PreSaveFcn=plecs('sl', 311);  NameChangeFcn=plecs('sl', 310);  DestroyFcn=plecs('sl', 307);  OpenFcn=plecs('sl', 302);  ErrorFcn=plerrorfcn
      mask Display: plot([0.1 0.9 0.9 0.1 0.1], [0.9 0.9 0.5 0.5 0.9])
  Sum : Sum  Inputs=|+-
  velocity regulator : Subsystem
  Te* (k) : Outport  PortDimensions=1
  wires:
  Sum/1 -> Scope4/1(1), velocity regulator/1(Err_v)
  w_rm (k)/1 -> Sum/2
  velocity regulator/1(Te*) -> Scope4/2(2), Te* (k)/1
  w_rm* (k)/1 -> Rate Limiter/1
  Rate Limiter/1 -> Sum/1

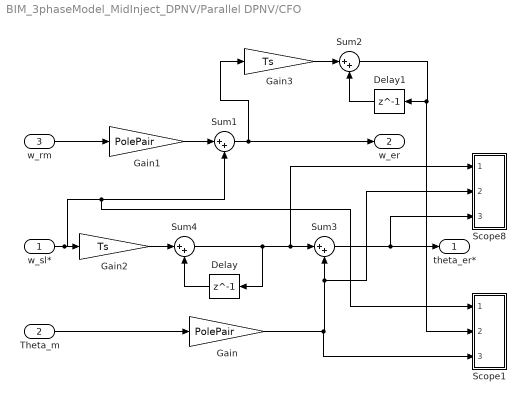
== system BIM_3phaseModel_MidInject_DPNV/Parallel DPNV/CFO ==
  w_sl* : Inport
  Theta_m : Inport  Port=2
  w_rm : Inport  Port=3
  Delay : Delay  DelayLength=1  InitialCondition=0  SampleTime=Ts
  Delay1 : Delay  DelayLength=1  InitialCondition=0  SampleTime=Ts
  Gain : Gain  Gain=PolePair
  Gain1 : Gain  Gain=PolePair
  Gain2 : Gain  Gain=Ts
  Gain3 : Gain  Gain=Ts
  Scope1 : Subsystem  LoadFcn=plecs('sl', 300);  InitFcn=plecs('sl', 314);  StartFcn=plecs('sl', 308);  StopFcn=plecs('sl', 309);  mask{Settings=<binary blob, 232 chars, not shown>}
      mask init:
      | plecs('sl', 315);
      settings: CopyFcn=plecs('sl', 303);  DeleteFcn=plecs('sl', 305);  UndoDeleteFcn=plecs('sl', 306);  PreSaveFcn=plecs('sl', 311);  NameChangeFcn=plecs('sl', 310);  DestroyFcn=plecs('sl', 307);  OpenFcn=plecs('sl', 302);  ErrorFcn=plerrorfcn
      mask Display: plot([0.1 0.9 0.9 0.1 0.1], [0.9 0.9 0.5 0.5 0.9])
  Scope8 : Subsystem  LoadFcn=plecs('sl', 300);  InitFcn=plecs('sl', 314);  StartFcn=plecs('sl', 308);  StopFcn=plecs('sl', 309);  mask{Settings=<binary blob, 232 chars, not shown>}
      mask init:
      | plecs('sl', 315);
      settings: CopyFcn=plecs('sl', 303);  DeleteFcn=plecs('sl', 305);  UndoDeleteFcn=plecs('sl', 306);  PreSaveFcn=plecs('sl', 311);  NameChangeFcn=plecs('sl', 310);  DestroyFcn=plecs('sl', 307);  OpenFcn=plecs('sl', 302);  ErrorFcn=plerrorfcn
      mask Display: plot([0.1 0.9 0.9 0.1 0.1], [0.9 0.9 0.5 0.5 0.9])
  Sum{1..4} (4 alike) : Sum  Inputs=|++
  theta_er* : Outport
  w_er : Outport  Port=2
  wires:
  Theta_m/1 -> Gain/1
  Sum4/1 -> Scope8/1(1), Sum3/1, Delay/1
  Sum3/1 -> Scope8/3(3), theta_er*/1
  w_sl*/1 -> Scope1/1(1), Sum1/2, Gain2/1
  Gain/1 -> Scope1/3(3), Scope8/2(2), Sum3/2
  Delay/1 -> Sum4/2
  Gain2/1 -> Sum4/1
  w_rm/1 -> Gain1/1
  Gain1/1 -> Sum1/1
  Delay1/1 -> Sum2/2
  Sum1/1 -> Gain3/1, w_er/1
  Gain3/1 -> Sum2/1
  Sum2/1 -> Scope1/2(2), Delay1/1

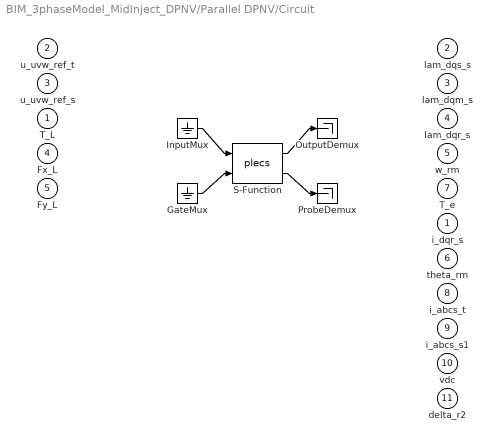
== system BIM_3phaseModel_MidInject_DPNV/Parallel DPNV/Circuit ==
  T_L : Inport  PortDimensions=1
  u_uvw_ref_t : Inport  Port=2  PortDimensions=3
  u_uvw_ref_s : Inport  Port=3  PortDimensions=3
  Fx_L : Inport  Port=4  PortDimensions=1
  Fy_L : Inport  Port=5  PortDimensions=1
  " GateMux " : Ground
  " InputMux " : Ground
  " OutputDemux " : Terminator
  " ProbeDemux " : Terminator
  " S-Function " : S-Function  FunctionName=plecs  SFunctionDeploymentMode=off  EnableBusSupport=off
  i_dqr_s : Outport  PortDimensions=3
  lam_dqs_s : Outport  Port=2  PortDimensions=2
  lam_dqm_s : Outport  Port=3  PortDimensions=2
  lam_dqr_s : Outport  Port=4  PortDimensions=2
  w_rm : Outport  Port=5  PortDimensions=1
  theta_rm : Outport  Port=6  PortDimensions=1
  T_e : Outport  Port=7  PortDimensions=1
  i_abcs_t : Outport  Port=8  PortDimensions=3
  i_abcs_s1 : Outport  Port=9  PortDimensions=3
  vdc : Outport  Port=10  PortDimensions=1
  delta_r2 : Outport  Port=11  PortDimensions=2
  wires:
  " InputMux "/1 -> " S-Function "/1
  " GateMux "/1 -> " S-Function "/2
  " S-Function "/1 -> " OutputDemux "/1
  " S-Function "/2 -> " ProbeDemux "/1
